simulink model "WaterTank_10Tanks_Model"  (R2013a)
settings: Solver=ode3  StartTime=0.0  StopTime=30.0  FixedStep=0.001  RelTol=1e-3
InitFcn:
  | initparametersDACADC
undefined symbols (not defined in the file): Ad, Bd, Cd, Dd, x0
libraries: commutil2 x1080, xpclib x142, etargetslib x140, dspnetwork x140, commcrc2 x20, simulink x1
(part 3 of 9)

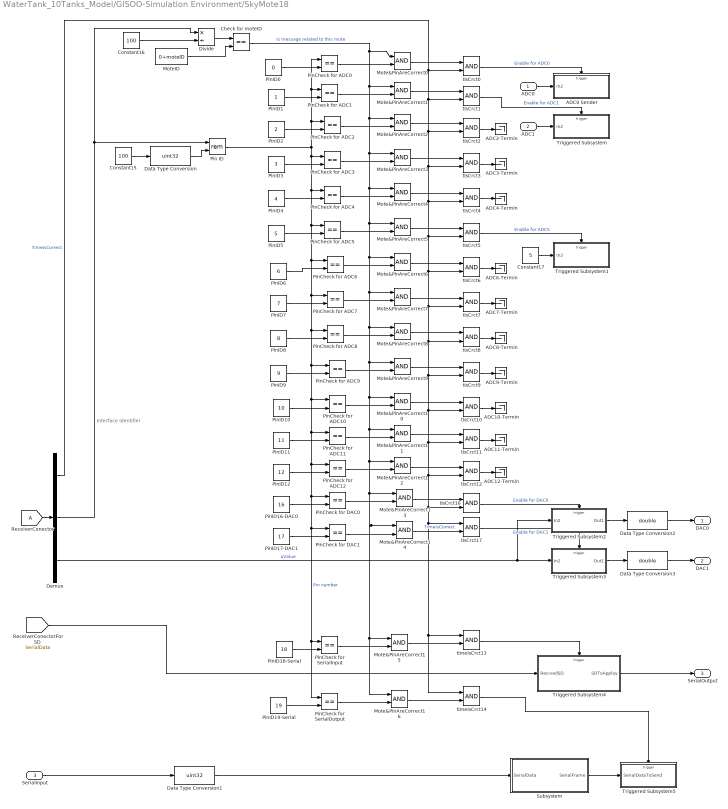
== system WaterTank_10Tanks_Model/GISOO-Simulation Environment/SkyMote18 ==
  note: Interface Identifier
  ADC0 : Inport
  ADC1 : Inport  Port=2
  SerialInput : Inport  Port=3
  ADC0 Sender : Subsystem  TreatAsAtomicUnit=on
  ADC10-Termin : Terminator
  ADC11-Termin : Terminator
  ADC12-Termin : Terminator
  ADC2-Termin : Terminator
  ADC3-Termin : Terminator
  ADC4-Termin : Terminator
  ADC6-Termin : Terminator
  ADC7-Termin : Terminator
  ADC8-Termin : Terminator
  ADC9-Termin : Terminator
  Check for moteID : RelationalOperator  Operator===  OutDataTypeStr=boolean
  Constant15 : Constant  Value=100
  Constant16 : Constant  Value=100
  Constant17 : Constant  Value=5
  Data Type Conversion : DataTypeConversion  OutDataTypeStr=uint32
  Data Type Conversion1 : DataTypeConversion  OutDataTypeStr=uint32
  Data Type Conversion2 : DataTypeConversion  OutDataTypeStr=double
  Data Type Conversion3 : DataTypeConversion  OutDataTypeStr=double
  Demux : Demux  Outputs=3
  Divide : Product  Inputs=*/  OutDataTypeStr=int32
  Mote&PinAreCorrect{0..16} (17 alike) : Logic  AllPortsSameDT=off  OutDataTypeStr=boolean
  MoteID : Constant  Value=0+moteID
  Pin ID : Math  Operator=rem  SaturateOnIntegerOverflow=on
  PinCheck for ADC{0..12} (13 alike) : RelationalOperator  Operator===  OutDataTypeStr=boolean
  PinCheck for DAC0 : RelationalOperator  Operator===  OutDataTypeStr=boolean
  PinCheck for DAC1 : RelationalOperator  Operator===  OutDataTypeStr=boolean
  PinCheck for SerialInput : RelationalOperator  Operator===  OutDataTypeStr=boolean
  PinCheck for SerialOutput : RelationalOperator  Operator===  OutDataTypeStr=boolean
  PinID0 : Constant  Value=0
  PinID1 : Constant
  PinID10 : Constant  Value=10
  PinID11 : Constant  Value=11
  PinID12 : Constant  Value=12
  PinID16-DAC0 : Constant  Value=16
  PinID17-DAC1 : Constant  Value=17
  PinID18-Serial : Constant  Value=18
  PinID19-Serial : Constant  Value=19
  PinID2 : Constant  Value=2
  PinID3 : Constant  Value=3
  PinID4 : Constant  Value=4
  PinID5 : Constant  Value=5
  PinID6 : Constant  Value=6
  PinID7 : Constant  Value=7
  PinID8 : Constant  Value=8
  PinID9 : Constant  Value=9
  Subsystem : Subsystem
  Triggered Subsystem : Subsystem  TreatAsAtomicUnit=on
  Triggered Subsystem1 : Subsystem  TreatAsAtomicUnit=on
  Triggered Subsystem2 : Subsystem  TreatAsAtomicUnit=on
  Triggered Subsystem3 : Subsystem  TreatAsAtomicUnit=on
  Triggered Subsystem4 : Subsystem  TreatAsAtomicUnit=on
  Triggered Subsystem5 : Subsystem  TreatAsAtomicUnit=on
  tIsCrct{0..12,16..17} (15 alike) : Logic  AllPortsSameDT=off  OutDataTypeStr=boolean
  timeIsCrct13 : Logic  AllPortsSameDT=off  OutDataTypeStr=boolean
  timeIsCrct14 : Logic  AllPortsSameDT=off  OutDataTypeStr=boolean
  DAC0 : Outport
  DAC1 : Outport  Port=2
  SerialOutput : Outport  Port=3
  wires:
  PinCheck for SerialInput/1 -> Mote&PinAreCorrect15/2
  Data Type Conversion1/1 -> Subsystem/1(SerialData)
  SerialInput/1 -> Data Type Conversion1/1
  timeIsCrct14/1 -> Triggered Subsystem5/Trigger
  Mote&PinAreCorrect16/1 -> timeIsCrct14/2
  PinCheck for SerialOutput/1 -> Mote&PinAreCorrect16/2
  PinID19-Serial/1 -> PinCheck for SerialOutput/2
  Check for moteID/1 -> Mote&PinAreCorrect0/1, Mote&PinAreCorrect2/1, Mote&PinAreCorrect3/1, Mote&PinAreCorrect4/1, Mote&PinAreCorrect5/1, Mote&PinAreCorrect6/1, Mote&PinAreCorrect7/1, Mote&PinAreCorrect8/1, Mote&PinAreCorrect9/1, Mote&PinAreCorrect10/1, Mote&PinAreCorrect11/1, Mote&PinAreCorrect12/1, Mote&PinAreCorrect15/1, Mote&PinAreCorrect16/1, Mote&PinAreCorrect14/1, Mote&PinAreCorrect13/1, Mote&PinAreCorrect1/1  "Is message related to this mote"
  Mote&PinAreCorrect15/1 -> timeIsCrct13/2
  Pin ID/1 -> PinCheck for ADC3/1, PinCheck for ADC4/1, PinCheck for ADC5/1, PinCheck for ADC6/1, PinCheck for ADC7/1, PinCheck for ADC8/1, PinCheck for ADC9/1, PinCheck for ADC10/1, PinCheck for ADC11/1, PinCheck for ADC12/1, PinCheck for DAC0/1, PinCheck for DAC1/1, PinCheck for SerialInput/1, PinCheck for SerialOutput/1, PinCheck for ADC2/1, PinCheck for ADC1/1, PinCheck for ADC0/1  "Pin number"
  tIsCrct12/1 -> ADC12-Termin/1
  Triggered Subsystem4/1(SDToApplay) -> SerialOutput/1
  Mote&PinAreCorrect14/1 -> tIsCrct17/2  "TimeIsCorrect"
  timeIsCrct13/1 -> Triggered Subsystem4/Trigger
  [SerialData] -> Triggered Subsystem4/1(RecivedSD)
  PinID18-Serial/1 -> PinCheck for SerialInput/2
  Demux/1 -> tIsCrct17/1, timeIsCrct13/1, timeIsCrct14/1, tIsCrct16/2, tIsCrct12/2, tIsCrct11/2, tIsCrct10/2, tIsCrct9/2, tIsCrct8/2, tIsCrct7/2, tIsCrct6/2, tIsCrct5/2, tIsCrct4/2, tIsCrct3/2, tIsCrct2/2, tIsCrct1/2, tIsCrct0/2  "TimeIsCorrect"
  Subsystem/1(SerialFrame) -> Triggered Subsystem5/1(SerialDataToSend)
  PinID17-DAC1/1 -> PinCheck for DAC1/2
  PinID16-DAC0/1 -> PinCheck for DAC0/2
  PinID12/1 -> PinCheck for ADC12/2
  PinID11/1 -> PinCheck for ADC11/2
  PinID9/1 -> PinCheck for ADC9/2
  PinID1/1 -> PinCheck for ADC1/2
  PinID10/1 -> PinCheck for ADC10/2
  PinID8/1 -> PinCheck for ADC8/2
  PinID7/1 -> PinCheck for ADC7/2
  PinID6/1 -> PinCheck for ADC6/2
  PinID5/1 -> PinCheck for ADC5/2
  PinID4/1 -> PinCheck for ADC4/2
  PinID3/1 -> PinCheck for ADC3/2
  PinID2/1 -> PinCheck for ADC2/2
  PinID0/1 -> PinCheck for ADC0/2
  PinCheck for ADC0/1 -> Mote&PinAreCorrect0/2
  PinCheck for ADC1/1 -> Mote&PinAreCorrect1/2
  PinCheck for ADC2/1 -> Mote&PinAreCorrect2/2
  PinCheck for ADC3/1 -> Mote&PinAreCorrect3/2
  PinCheck for ADC4/1 -> Mote&PinAreCorrect4/2
  PinCheck for ADC5/1 -> Mote&PinAreCorrect5/2
  PinCheck for ADC6/1 -> Mote&PinAreCorrect6/2
  PinCheck for ADC7/1 -> Mote&PinAreCorrect7/2
  PinCheck for ADC8/1 -> Mote&PinAreCorrect8/2
  PinCheck for ADC9/1 -> Mote&PinAreCorrect9/2
  PinCheck for ADC10/1 -> Mote&PinAreCorrect10/2
  PinCheck for ADC11/1 -> Mote&PinAreCorrect11/2
  PinCheck for ADC12/1 -> Mote&PinAreCorrect12/2
  PinCheck for DAC0/1 -> Mote&PinAreCorrect13/2
  PinCheck for DAC1/1 -> Mote&PinAreCorrect14/2
  Constant16/1 -> Divide/2
  Divide/1 -> Check for moteID/1
  MoteID/1 -> Check for moteID/2
  Mote&PinAreCorrect13/1 -> tIsCrct16/1
  Mote&PinAreCorrect12/1 -> tIsCrct12/1
  Mote&PinAreCorrect8/1 -> tIsCrct8/1
  Mote&PinAreCorrect7/1 -> tIsCrct7/1
  Mote&PinAreCorrect6/1 -> tIsCrct6/1
  Mote&PinAreCorrect4/1 -> tIsCrct4/1
  Mote&PinAreCorrect3/1 -> tIsCrct3/1
  Constant15/1 -> Data Type Conversion/1
  Data Type Conversion/1 -> Pin ID/2
  tIsCrct16/1 -> Triggered Subsystem2/Trigger  "Enable for DAC0"
  tIsCrct17/1 -> Triggered Subsystem3/Trigger  "Enable for DAC1"
  [A] -> Demux/1
  Demux/3 -> Triggered Subsystem3/1(In2), Triggered Subsystem2/1(In2)  "uValue"
  ADC0/1 -> ADC0 Sender/1(In2)
  Demux/2 -> Divide/1, Pin ID/1
  Data Type Conversion2/1 -> DAC0/1
  Triggered Subsystem2/1(Out1) -> Data Type Conversion2/1
  Data Type Conversion3/1 -> DAC1/1
  Triggered Subsystem3/1(Out1) -> Data Type Conversion3/1
  Constant17/1 -> Triggered Subsystem1/1(In2)
  Mote&PinAreCorrect0/1 -> tIsCrct0/1
  tIsCrct0/1 -> ADC0 Sender/Trigger  "Enable for ADC0"
  ADC1/1 -> Triggered Subsystem/1(In2)
  Mote&PinAreCorrect1/1 -> tIsCrct1/1
  tIsCrct1/1 -> Triggered Subsystem/Trigger  "Enable for ADC1"
  tIsCrct2/1 -> ADC2-Termin/1
  Mote&PinAreCorrect2/1 -> tIsCrct2/1
  tIsCrct3/1 -> ADC3-Termin/1
  tIsCrct4/1 -> ADC4-Termin/1
  tIsCrct6/1 -> ADC6-Termin/1
  Mote&PinAreCorrect5/1 -> tIsCrct5/1
  tIsCrct5/1 -> Triggered Subsystem1/Trigger  "Enable for ADC5"
  tIsCrct7/1 -> ADC7-Termin/1
  tIsCrct8/1 -> ADC8-Termin/1
  tIsCrct9/1 -> ADC9-Termin/1
  Mote&PinAreCorrect9/1 -> tIsCrct9/1
  tIsCrct10/1 -> ADC10-Termin/1
  Mote&PinAreCorrect10/1 -> tIsCrct10/1
  tIsCrct11/1 -> ADC11-Termin/1
  Mote&PinAreCorrect11/1 -> tIsCrct11/1

== system WaterTank_10Tanks_Model/GISOO-Simulation Environment/SkyMote19 ==
  note: Interface Identifier
  ADC0 : Inport
  ADC1 : Inport  Port=2
  SerialInput : Inport  Port=3
  ADC0 Sender : Subsystem  TreatAsAtomicUnit=on
  ADC10-Termin : Terminator
  ADC11-Termin : Terminator
  ADC12-Termin : Terminator
  ADC2-Termin : Terminator
  ADC3-Termin : Terminator
  ADC4-Termin : Terminator
  ADC6-Termin : Terminator
  ADC7-Termin : Terminator
  ADC8-Termin : Terminator
  ADC9-Termin : Terminator
  Check for moteID : RelationalOperator  Operator===  OutDataTypeStr=boolean
  Constant15 : Constant  Value=100
  Constant16 : Constant  Value=100
  Constant17 : Constant  Value=5
  Data Type Conversion : DataTypeConversion  OutDataTypeStr=uint32
  Data Type Conversion1 : DataTypeConversion  OutDataTypeStr=uint32
  Data Type Conversion2 : DataTypeConversion  OutDataTypeStr=double
  Data Type Conversion3 : DataTypeConversion  OutDataTypeStr=double
  Demux : Demux  Outputs=3
  Divide : Product  Inputs=*/  OutDataTypeStr=int32
  Mote&PinAreCorrect{0..16} (17 alike) : Logic  AllPortsSameDT=off  OutDataTypeStr=boolean
  MoteID : Constant  Value=0+moteID
  Pin ID : Math  Operator=rem  SaturateOnIntegerOverflow=on
  PinCheck for ADC{0..12} (13 alike) : RelationalOperator  Operator===  OutDataTypeStr=boolean
  PinCheck for DAC0 : RelationalOperator  Operator===  OutDataTypeStr=boolean
  PinCheck for DAC1 : RelationalOperator  Operator===  OutDataTypeStr=boolean
  PinCheck for SerialInput : RelationalOperator  Operator===  OutDataTypeStr=boolean
  PinCheck for SerialOutput : RelationalOperator  Operator===  OutDataTypeStr=boolean
  PinID0 : Constant  Value=0
  PinID1 : Constant
  PinID10 : Constant  Value=10
  PinID11 : Constant  Value=11
  PinID12 : Constant  Value=12
  PinID16-DAC0 : Constant  Value=16
  PinID17-DAC1 : Constant  Value=17
  PinID18-Serial : Constant  Value=18
  PinID19-Serial : Constant  Value=19
  PinID2 : Constant  Value=2
  PinID3 : Constant  Value=3
  PinID4 : Constant  Value=4
  PinID5 : Constant  Value=5
  PinID6 : Constant  Value=6
  PinID7 : Constant  Value=7
  PinID8 : Constant  Value=8
  PinID9 : Constant  Value=9
  Subsystem : Subsystem
  Triggered Subsystem : Subsystem  TreatAsAtomicUnit=on
  Triggered Subsystem1 : Subsystem  TreatAsAtomicUnit=on
  Triggered Subsystem2 : Subsystem  TreatAsAtomicUnit=on
  Triggered Subsystem3 : Subsystem  TreatAsAtomicUnit=on
  Triggered Subsystem4 : Subsystem  TreatAsAtomicUnit=on
  Triggered Subsystem5 : Subsystem  TreatAsAtomicUnit=on
  tIsCrct{0..12,16..17} (15 alike) : Logic  AllPortsSameDT=off  OutDataTypeStr=boolean
  timeIsCrct13 : Logic  AllPortsSameDT=off  OutDataTypeStr=boolean
  timeIsCrct14 : Logic  AllPortsSameDT=off  OutDataTypeStr=boolean
  DAC0 : Outport
  DAC1 : Outport  Port=2
  SerialOutput : Outport  Port=3
  wires:
  Mote&PinAreCorrect11/1 -> tIsCrct11/1
  tIsCrct11/1 -> ADC11-Termin/1
  Mote&PinAreCorrect10/1 -> tIsCrct10/1
  tIsCrct10/1 -> ADC10-Termin/1
  Mote&PinAreCorrect9/1 -> tIsCrct9/1
  tIsCrct9/1 -> ADC9-Termin/1
  tIsCrct8/1 -> ADC8-Termin/1
  tIsCrct7/1 -> ADC7-Termin/1
  tIsCrct5/1 -> Triggered Subsystem1/Trigger  "Enable for ADC5"
  Mote&PinAreCorrect5/1 -> tIsCrct5/1
  tIsCrct6/1 -> ADC6-Termin/1
  tIsCrct4/1 -> ADC4-Termin/1
  tIsCrct3/1 -> ADC3-Termin/1
  Mote&PinAreCorrect2/1 -> tIsCrct2/1
  tIsCrct2/1 -> ADC2-Termin/1
  tIsCrct1/1 -> Triggered Subsystem/Trigger  "Enable for ADC1"
  Mote&PinAreCorrect1/1 -> tIsCrct1/1
  ADC1/1 -> Triggered Subsystem/1(In2)
  tIsCrct0/1 -> ADC0 Sender/Trigger  "Enable for ADC0"
  Mote&PinAreCorrect0/1 -> tIsCrct0/1
  Constant17/1 -> Triggered Subsystem1/1(In2)
  Triggered Subsystem3/1(Out1) -> Data Type Conversion3/1
  Data Type Conversion3/1 -> DAC1/1
  Triggered Subsystem2/1(Out1) -> Data Type Conversion2/1
  Data Type Conversion2/1 -> DAC0/1
  Demux/2 -> Pin ID/1, Divide/1
  ADC0/1 -> ADC0 Sender/1(In2)
  Demux/3 -> Triggered Subsystem2/1(In2), Triggered Subsystem3/1(In2)  "uValue"
  [A] -> Demux/1
  tIsCrct17/1 -> Triggered Subsystem3/Trigger  "Enable for DAC1"
  tIsCrct16/1 -> Triggered Subsystem2/Trigger  "Enable for DAC0"
  Data Type Conversion/1 -> Pin ID/2
  Constant15/1 -> Data Type Conversion/1
  Mote&PinAreCorrect3/1 -> tIsCrct3/1
  Mote&PinAreCorrect4/1 -> tIsCrct4/1
  Mote&PinAreCorrect6/1 -> tIsCrct6/1
  Mote&PinAreCorrect7/1 -> tIsCrct7/1
  Mote&PinAreCorrect8/1 -> tIsCrct8/1
  Mote&PinAreCorrect12/1 -> tIsCrct12/1
  Mote&PinAreCorrect13/1 -> tIsCrct16/1
  MoteID/1 -> Check for moteID/2
  Divide/1 -> Check for moteID/1
  Constant16/1 -> Divide/2
  PinCheck for DAC1/1 -> Mote&PinAreCorrect14/2
  PinCheck for DAC0/1 -> Mote&PinAreCorrect13/2
  PinCheck for ADC12/1 -> Mote&PinAreCorrect12/2
  PinCheck for ADC11/1 -> Mote&PinAreCorrect11/2
  PinCheck for ADC10/1 -> Mote&PinAreCorrect10/2
  PinCheck for ADC9/1 -> Mote&PinAreCorrect9/2
  PinCheck for ADC8/1 -> Mote&PinAreCorrect8/2
  PinCheck for ADC7/1 -> Mote&PinAreCorrect7/2
  PinCheck for ADC6/1 -> Mote&PinAreCorrect6/2
  PinCheck for ADC5/1 -> Mote&PinAreCorrect5/2
  PinCheck for ADC4/1 -> Mote&PinAreCorrect4/2
  PinCheck for ADC3/1 -> Mote&PinAreCorrect3/2
  PinCheck for ADC2/1 -> Mote&PinAreCorrect2/2
  PinCheck for ADC1/1 -> Mote&PinAreCorrect1/2
  PinCheck for ADC0/1 -> Mote&PinAreCorrect0/2
  PinID0/1 -> PinCheck for ADC0/2
  PinID2/1 -> PinCheck for ADC2/2
  PinID3/1 -> PinCheck for ADC3/2
  PinID4/1 -> PinCheck for ADC4/2
  PinID5/1 -> PinCheck for ADC5/2
  PinID6/1 -> PinCheck for ADC6/2
  PinID7/1 -> PinCheck for ADC7/2
  PinID8/1 -> PinCheck for ADC8/2
  PinID10/1 -> PinCheck for ADC10/2
  PinID1/1 -> PinCheck for ADC1/2
  PinID9/1 -> PinCheck for ADC9/2
  PinID11/1 -> PinCheck for ADC11/2
  PinID12/1 -> PinCheck for ADC12/2
  PinID16-DAC0/1 -> PinCheck for DAC0/2
  PinID17-DAC1/1 -> PinCheck for DAC1/2
  Subsystem/1(SerialFrame) -> Triggered Subsystem5/1(SerialDataToSend)
  Demux/1 -> tIsCrct0/2, tIsCrct1/2, tIsCrct2/2, tIsCrct3/2, tIsCrct4/2, tIsCrct5/2, tIsCrct6/2, tIsCrct7/2, tIsCrct8/2, tIsCrct9/2, tIsCrct10/2, tIsCrct11/2, tIsCrct12/2, tIsCrct16/2, timeIsCrct14/1, timeIsCrct13/1, tIsCrct17/1  "TimeIsCorrect"
  PinID18-Serial/1 -> PinCheck for SerialInput/2
  [SerialData] -> Triggered Subsystem4/1(RecivedSD)
  timeIsCrct13/1 -> Triggered Subsystem4/Trigger
  Mote&PinAreCorrect14/1 -> tIsCrct17/2  "TimeIsCorrect"
  Triggered Subsystem4/1(SDToApplay) -> SerialOutput/1
  tIsCrct12/1 -> ADC12-Termin/1
  Pin ID/1 -> PinCheck for ADC0/1, PinCheck for ADC1/1, PinCheck for ADC2/1, PinCheck for SerialOutput/1, PinCheck for SerialInput/1, PinCheck for DAC1/1, PinCheck for DAC0/1, PinCheck for ADC12/1, PinCheck for ADC11/1, PinCheck for ADC10/1, PinCheck for ADC9/1, PinCheck for ADC8/1, PinCheck for ADC7/1, PinCheck for ADC6/1, PinCheck for ADC5/1, PinCheck for ADC4/1, PinCheck for ADC3/1  "Pin number"
  Mote&PinAreCorrect15/1 -> timeIsCrct13/2
  Check for moteID/1 -> Mote&PinAreCorrect1/1, Mote&PinAreCorrect13/1, Mote&PinAreCorrect14/1, Mote&PinAreCorrect16/1, Mote&PinAreCorrect15/1, Mote&PinAreCorrect12/1, Mote&PinAreCorrect11/1, Mote&PinAreCorrect10/1, Mote&PinAreCorrect9/1, Mote&PinAreCorrect8/1, Mote&PinAreCorrect7/1, Mote&PinAreCorrect6/1, Mote&PinAreCorrect5/1, Mote&PinAreCorrect4/1, Mote&PinAreCorrect3/1, Mote&PinAreCorrect2/1, Mote&PinAreCorrect0/1  "Is message related to this mote"
  PinID19-Serial/1 -> PinCheck for SerialOutput/2
  PinCheck for SerialOutput/1 -> Mote&PinAreCorrect16/2
  Mote&PinAreCorrect16/1 -> timeIsCrct14/2
  timeIsCrct14/1 -> Triggered Subsystem5/Trigger
  SerialInput/1 -> Data Type Conversion1/1
  Data Type Conversion1/1 -> Subsystem/1(SerialData)
  PinCheck for SerialInput/1 -> Mote&PinAreCorrect15/2

== system WaterTank_10Tanks_Model/GISOO-Simulation Environment/SkyMote2 ==
  note: Interface Identifier
  ADC0 : Inport
  ADC1 : Inport  Port=2
  SerialInput : Inport  Port=3
  ADC0 Sender : Subsystem  TreatAsAtomicUnit=on
  ADC10-Termin : Terminator
  ADC11-Termin : Terminator
  ADC12-Termin : Terminator
  ADC2-Termin : Terminator
  ADC3-Termin : Terminator
  ADC4-Termin : Terminator
  ADC6-Termin : Terminator
  ADC7-Termin : Terminator
  ADC8-Termin : Terminator
  ADC9-Termin : Terminator
  Check for moteID : RelationalOperator  Operator===  OutDataTypeStr=boolean
  Constant15 : Constant  Value=100
  Constant16 : Constant  Value=100
  Constant17 : Constant  Value=5
  Data Type Conversion : DataTypeConversion  OutDataTypeStr=uint32
  Data Type Conversion1 : DataTypeConversion  OutDataTypeStr=uint32
  Data Type Conversion2 : DataTypeConversion  OutDataTypeStr=double
  Data Type Conversion3 : DataTypeConversion  OutDataTypeStr=double
  Demux : Demux  Outputs=3
  Divide : Product  Inputs=*/  OutDataTypeStr=int32
  Mote&PinAreCorrect{0..16} (17 alike) : Logic  AllPortsSameDT=off  OutDataTypeStr=boolean
  MoteID : Constant  Value=0+moteID
  Pin ID : Math  Operator=rem  SaturateOnIntegerOverflow=on
  PinCheck for ADC{0..12} (13 alike) : RelationalOperator  Operator===  OutDataTypeStr=boolean
  PinCheck for DAC0 : RelationalOperator  Operator===  OutDataTypeStr=boolean
  PinCheck for DAC1 : RelationalOperator  Operator===  OutDataTypeStr=boolean
  PinCheck for SerialInput : RelationalOperator  Operator===  OutDataTypeStr=boolean
  PinCheck for SerialOutput : RelationalOperator  Operator===  OutDataTypeStr=boolean
  PinID0 : Constant  Value=0
  PinID1 : Constant
  PinID10 : Constant  Value=10
  PinID11 : Constant  Value=11
  PinID12 : Constant  Value=12
  PinID16-DAC0 : Constant  Value=16
  PinID17-DAC1 : Constant  Value=17
  PinID18-Serial : Constant  Value=18
  PinID19-Serial : Constant  Value=19
  PinID2 : Constant  Value=2
  PinID3 : Constant  Value=3
  PinID4 : Constant  Value=4
  PinID5 : Constant  Value=5
  PinID6 : Constant  Value=6
  PinID7 : Constant  Value=7
  PinID8 : Constant  Value=8
  PinID9 : Constant  Value=9
  Subsystem : Subsystem
  Triggered Subsystem : Subsystem  TreatAsAtomicUnit=on
  Triggered Subsystem1 : Subsystem  TreatAsAtomicUnit=on
  Triggered Subsystem2 : Subsystem  TreatAsAtomicUnit=on
  Triggered Subsystem3 : Subsystem  TreatAsAtomicUnit=on
  Triggered Subsystem4 : Subsystem  TreatAsAtomicUnit=on
  Triggered Subsystem5 : Subsystem  TreatAsAtomicUnit=on
  tIsCrct{0..12,16..17} (15 alike) : Logic  AllPortsSameDT=off  OutDataTypeStr=boolean
  timeIsCrct13 : Logic  AllPortsSameDT=off  OutDataTypeStr=boolean
  timeIsCrct14 : Logic  AllPortsSameDT=off  OutDataTypeStr=boolean
  DAC0 : Outport
  DAC1 : Outport  Port=2
  SerialOutput : Outport  Port=3
  wires:
  PinCheck for SerialInput/1 -> Mote&PinAreCorrect15/2
  Data Type Conversion1/1 -> Subsystem/1(SerialData)
  SerialInput/1 -> Data Type Conversion1/1
  timeIsCrct14/1 -> Triggered Subsystem5/Trigger
  Mote&PinAreCorrect16/1 -> timeIsCrct14/2
  PinCheck for SerialOutput/1 -> Mote&PinAreCorrect16/2
  PinID19-Serial/1 -> PinCheck for SerialOutput/2
  Check for moteID/1 -> Mote&PinAreCorrect0/1, Mote&PinAreCorrect2/1, Mote&PinAreCorrect3/1, Mote&PinAreCorrect4/1, Mote&PinAreCorrect5/1, Mote&PinAreCorrect6/1, Mote&PinAreCorrect7/1, Mote&PinAreCorrect8/1, Mote&PinAreCorrect9/1, Mote&PinAreCorrect10/1, Mote&PinAreCorrect11/1, Mote&PinAreCorrect12/1, Mote&PinAreCorrect15/1, Mote&PinAreCorrect16/1, Mote&PinAreCorrect14/1, Mote&PinAreCorrect13/1, Mote&PinAreCorrect1/1  "Is message related to this mote"
  Mote&PinAreCorrect15/1 -> timeIsCrct13/2
  Pin ID/1 -> PinCheck for ADC3/1, PinCheck for ADC4/1, PinCheck for ADC5/1, PinCheck for ADC6/1, PinCheck for ADC7/1, PinCheck for ADC8/1, PinCheck for ADC9/1, PinCheck for ADC10/1, PinCheck for ADC11/1, PinCheck for ADC12/1, PinCheck for DAC0/1, PinCheck for DAC1/1, PinCheck for SerialInput/1, PinCheck for SerialOutput/1, PinCheck for ADC2/1, PinCheck for ADC1/1, PinCheck for ADC0/1  "Pin number"
  tIsCrct12/1 -> ADC12-Termin/1
  Triggered Subsystem4/1(SDToApplay) -> SerialOutput/1
  Mote&PinAreCorrect14/1 -> tIsCrct17/2  "TimeIsCorrect"
  timeIsCrct13/1 -> Triggered Subsystem4/Trigger
  [SerialData] -> Triggered Subsystem4/1(RecivedSD)
  PinID18-Serial/1 -> PinCheck for SerialInput/2
  Demux/1 -> tIsCrct17/1, timeIsCrct13/1, timeIsCrct14/1, tIsCrct16/2, tIsCrct12/2, tIsCrct11/2, tIsCrct10/2, tIsCrct9/2, tIsCrct8/2, tIsCrct7/2, tIsCrct6/2, tIsCrct5/2, tIsCrct4/2, tIsCrct3/2, tIsCrct2/2, tIsCrct1/2, tIsCrct0/2  "TimeIsCorrect"
  Subsystem/1(SerialFrame) -> Triggered Subsystem5/1(SerialDataToSend)
  PinID17-DAC1/1 -> PinCheck for DAC1/2
  PinID16-DAC0/1 -> PinCheck for DAC0/2
  PinID12/1 -> PinCheck for ADC12/2
  PinID11/1 -> PinCheck for ADC11/2
  PinID9/1 -> PinCheck for ADC9/2
  PinID1/1 -> PinCheck for ADC1/2
  PinID10/1 -> PinCheck for ADC10/2
  PinID8/1 -> PinCheck for ADC8/2
  PinID7/1 -> PinCheck for ADC7/2
  PinID6/1 -> PinCheck for ADC6/2
  PinID5/1 -> PinCheck for ADC5/2
  PinID4/1 -> PinCheck for ADC4/2
  PinID3/1 -> PinCheck for ADC3/2
  PinID2/1 -> PinCheck for ADC2/2
  PinID0/1 -> PinCheck for ADC0/2
  PinCheck for ADC0/1 -> Mote&PinAreCorrect0/2
  PinCheck for ADC1/1 -> Mote&PinAreCorrect1/2
  PinCheck for ADC2/1 -> Mote&PinAreCorrect2/2
  PinCheck for ADC3/1 -> Mote&PinAreCorrect3/2
  PinCheck for ADC4/1 -> Mote&PinAreCorrect4/2
  PinCheck for ADC5/1 -> Mote&PinAreCorrect5/2
  PinCheck for ADC6/1 -> Mote&PinAreCorrect6/2
  PinCheck for ADC7/1 -> Mote&PinAreCorrect7/2
  PinCheck for ADC8/1 -> Mote&PinAreCorrect8/2
  PinCheck for ADC9/1 -> Mote&PinAreCorrect9/2
  PinCheck for ADC10/1 -> Mote&PinAreCorrect10/2
  PinCheck for ADC11/1 -> Mote&PinAreCorrect11/2
  PinCheck for ADC12/1 -> Mote&PinAreCorrect12/2
  PinCheck for DAC0/1 -> Mote&PinAreCorrect13/2
  PinCheck for DAC1/1 -> Mote&PinAreCorrect14/2
  Constant16/1 -> Divide/2
  Divide/1 -> Check for moteID/1
  MoteID/1 -> Check for moteID/2
  Mote&PinAreCorrect13/1 -> tIsCrct16/1
  Mote&PinAreCorrect12/1 -> tIsCrct12/1
  Mote&PinAreCorrect8/1 -> tIsCrct8/1
  Mote&PinAreCorrect7/1 -> tIsCrct7/1
  Mote&PinAreCorrect6/1 -> tIsCrct6/1
  Mote&PinAreCorrect4/1 -> tIsCrct4/1
  Mote&PinAreCorrect3/1 -> tIsCrct3/1
  Constant15/1 -> Data Type Conversion/1
  Data Type Conversion/1 -> Pin ID/2
  tIsCrct16/1 -> Triggered Subsystem2/Trigger  "Enable for DAC0"
  tIsCrct17/1 -> Triggered Subsystem3/Trigger  "Enable for DAC1"
  [A] -> Demux/1
  Demux/3 -> Triggered Subsystem3/1(In2), Triggered Subsystem2/1(In2)  "uValue"
  ADC0/1 -> ADC0 Sender/1(In2)
  Demux/2 -> Divide/1, Pin ID/1
  Data Type Conversion2/1 -> DAC0/1
  Triggered Subsystem2/1(Out1) -> Data Type Conversion2/1
  Data Type Conversion3/1 -> DAC1/1
  Triggered Subsystem3/1(Out1) -> Data Type Conversion3/1
  Constant17/1 -> Triggered Subsystem1/1(In2)
  Mote&PinAreCorrect0/1 -> tIsCrct0/1
  tIsCrct0/1 -> ADC0 Sender/Trigger  "Enable for ADC0"
  ADC1/1 -> Triggered Subsystem/1(In2)
  Mote&PinAreCorrect1/1 -> tIsCrct1/1
  tIsCrct1/1 -> Triggered Subsystem/Trigger  "Enable for ADC1"
  tIsCrct2/1 -> ADC2-Termin/1
  Mote&PinAreCorrect2/1 -> tIsCrct2/1
  tIsCrct3/1 -> ADC3-Termin/1
  tIsCrct4/1 -> ADC4-Termin/1
  tIsCrct6/1 -> ADC6-Termin/1
  Mote&PinAreCorrect5/1 -> tIsCrct5/1
  tIsCrct5/1 -> Triggered Subsystem1/Trigger  "Enable for ADC5"
  tIsCrct7/1 -> ADC7-Termin/1
  tIsCrct8/1 -> ADC8-Termin/1
  tIsCrct9/1 -> ADC9-Termin/1
  Mote&PinAreCorrect9/1 -> tIsCrct9/1
  tIsCrct10/1 -> ADC10-Termin/1
  Mote&PinAreCorrect10/1 -> tIsCrct10/1
  tIsCrct11/1 -> ADC11-Termin/1
  Mote&PinAreCorrect11/1 -> tIsCrct11/1

== system WaterTank_10Tanks_Model/GISOO-Simulation Environment/SkyMote3 ==
  note: Interface Identifier
  ADC0 : Inport
  ADC1 : Inport  Port=2
  SerialInput : Inport  Port=3
  ADC0 Sender : Subsystem  TreatAsAtomicUnit=on
  ADC10-Termin : Terminator
  ADC11-Termin : Terminator
  ADC12-Termin : Terminator
  ADC2-Termin : Terminator
  ADC3-Termin : Terminator
  ADC4-Termin : Terminator
  ADC6-Termin : Terminator
  ADC7-Termin : Terminator
  ADC8-Termin : Terminator
  ADC9-Termin : Terminator
  Check for moteID : RelationalOperator  Operator===  OutDataTypeStr=boolean
  Constant15 : Constant  Value=100
  Constant16 : Constant  Value=100
  Constant17 : Constant  Value=5
  Data Type Conversion : DataTypeConversion  OutDataTypeStr=uint32
  Data Type Conversion1 : DataTypeConversion  OutDataTypeStr=uint32
  Data Type Conversion2 : DataTypeConversion  OutDataTypeStr=double
  Data Type Conversion3 : DataTypeConversion  OutDataTypeStr=double
  Demux : Demux  Outputs=3
  Divide : Product  Inputs=*/  OutDataTypeStr=int32
  Mote&PinAreCorrect{0..16} (17 alike) : Logic  AllPortsSameDT=off  OutDataTypeStr=boolean
  MoteID : Constant  Value=0+moteID
  Pin ID : Math  Operator=rem  SaturateOnIntegerOverflow=on
  PinCheck for ADC{0..12} (13 alike) : RelationalOperator  Operator===  OutDataTypeStr=boolean
  PinCheck for DAC0 : RelationalOperator  Operator===  OutDataTypeStr=boolean
  PinCheck for DAC1 : RelationalOperator  Operator===  OutDataTypeStr=boolean
  PinCheck for SerialInput : RelationalOperator  Operator===  OutDataTypeStr=boolean
  PinCheck for SerialOutput : RelationalOperator  Operator===  OutDataTypeStr=boolean
  PinID0 : Constant  Value=0
  PinID1 : Constant
  PinID10 : Constant  Value=10
  PinID11 : Constant  Value=11
  PinID12 : Constant  Value=12
  PinID16-DAC0 : Constant  Value=16
  PinID17-DAC1 : Constant  Value=17
  PinID18-Serial : Constant  Value=18
  PinID19-Serial : Constant  Value=19
  PinID2 : Constant  Value=2
  PinID3 : Constant  Value=3
  PinID4 : Constant  Value=4
  PinID5 : Constant  Value=5
  PinID6 : Constant  Value=6
  PinID7 : Constant  Value=7
  PinID8 : Constant  Value=8
  PinID9 : Constant  Value=9
  Subsystem : Subsystem
  Triggered Subsystem : Subsystem  TreatAsAtomicUnit=on
  Triggered Subsystem1 : Subsystem  TreatAsAtomicUnit=on
  Triggered Subsystem2 : Subsystem  TreatAsAtomicUnit=on
  Triggered Subsystem3 : Subsystem  TreatAsAtomicUnit=on
  Triggered Subsystem4 : Subsystem  TreatAsAtomicUnit=on
  Triggered Subsystem5 : Subsystem  TreatAsAtomicUnit=on
  tIsCrct{0..12,16..17} (15 alike) : Logic  AllPortsSameDT=off  OutDataTypeStr=boolean
  timeIsCrct13 : Logic  AllPortsSameDT=off  OutDataTypeStr=boolean
  timeIsCrct14 : Logic  AllPortsSameDT=off  OutDataTypeStr=boolean
  DAC0 : Outport
  DAC1 : Outport  Port=2
  SerialOutput : Outport  Port=3
  wires:
  Mote&PinAreCorrect11/1 -> tIsCrct11/1
  tIsCrct11/1 -> ADC11-Termin/1
  Mote&PinAreCorrect10/1 -> tIsCrct10/1
  tIsCrct10/1 -> ADC10-Termin/1
  Mote&PinAreCorrect9/1 -> tIsCrct9/1
  tIsCrct9/1 -> ADC9-Termin/1
  tIsCrct8/1 -> ADC8-Termin/1
  tIsCrct7/1 -> ADC7-Termin/1
  tIsCrct5/1 -> Triggered Subsystem1/Trigger  "Enable for ADC5"
  Mote&PinAreCorrect5/1 -> tIsCrct5/1
  tIsCrct6/1 -> ADC6-Termin/1
  tIsCrct4/1 -> ADC4-Termin/1
  tIsCrct3/1 -> ADC3-Termin/1
  Mote&PinAreCorrect2/1 -> tIsCrct2/1
  tIsCrct2/1 -> ADC2-Termin/1
  tIsCrct1/1 -> Triggered Subsystem/Trigger  "Enable for ADC1"
  Mote&PinAreCorrect1/1 -> tIsCrct1/1
  ADC1/1 -> Triggered Subsystem/1(In2)
  tIsCrct0/1 -> ADC0 Sender/Trigger  "Enable for ADC0"
  Mote&PinAreCorrect0/1 -> tIsCrct0/1
  Constant17/1 -> Triggered Subsystem1/1(In2)
  Triggered Subsystem3/1(Out1) -> Data Type Conversion3/1
  Data Type Conversion3/1 -> DAC1/1
  Triggered Subsystem2/1(Out1) -> Data Type Conversion2/1
  Data Type Conversion2/1 -> DAC0/1
  Demux/2 -> Pin ID/1, Divide/1
  ADC0/1 -> ADC0 Sender/1(In2)
  Demux/3 -> Triggered Subsystem2/1(In2), Triggered Subsystem3/1(In2)  "uValue"
  [A] -> Demux/1
  tIsCrct17/1 -> Triggered Subsystem3/Trigger  "Enable for DAC1"
  tIsCrct16/1 -> Triggered Subsystem2/Trigger  "Enable for DAC0"
  Data Type Conversion/1 -> Pin ID/2
  Constant15/1 -> Data Type Conversion/1
  Mote&PinAreCorrect3/1 -> tIsCrct3/1
  Mote&PinAreCorrect4/1 -> tIsCrct4/1
  Mote&PinAreCorrect6/1 -> tIsCrct6/1
  Mote&PinAreCorrect7/1 -> tIsCrct7/1
  Mote&PinAreCorrect8/1 -> tIsCrct8/1
  Mote&PinAreCorrect12/1 -> tIsCrct12/1
  Mote&PinAreCorrect13/1 -> tIsCrct16/1
  MoteID/1 -> Check for moteID/2
  Divide/1 -> Check for moteID/1
  Constant16/1 -> Divide/2
  PinCheck for DAC1/1 -> Mote&PinAreCorrect14/2
  PinCheck for DAC0/1 -> Mote&PinAreCorrect13/2
  PinCheck for ADC12/1 -> Mote&PinAreCorrect12/2
  PinCheck for ADC11/1 -> Mote&PinAreCorrect11/2
  PinCheck for ADC10/1 -> Mote&PinAreCorrect10/2
  PinCheck for ADC9/1 -> Mote&PinAreCorrect9/2
  PinCheck for ADC8/1 -> Mote&PinAreCorrect8/2
  PinCheck for ADC7/1 -> Mote&PinAreCorrect7/2
  PinCheck for ADC6/1 -> Mote&PinAreCorrect6/2
  PinCheck for ADC5/1 -> Mote&PinAreCorrect5/2
  PinCheck for ADC4/1 -> Mote&PinAreCorrect4/2
  PinCheck for ADC3/1 -> Mote&PinAreCorrect3/2
  PinCheck for ADC2/1 -> Mote&PinAreCorrect2/2
  PinCheck for ADC1/1 -> Mote&PinAreCorrect1/2
  PinCheck for ADC0/1 -> Mote&PinAreCorrect0/2
  PinID0/1 -> PinCheck for ADC0/2
  PinID2/1 -> PinCheck for ADC2/2
  PinID3/1 -> PinCheck for ADC3/2
  PinID4/1 -> PinCheck for ADC4/2
  PinID5/1 -> PinCheck for ADC5/2
  PinID6/1 -> PinCheck for ADC6/2
  PinID7/1 -> PinCheck for ADC7/2
  PinID8/1 -> PinCheck for ADC8/2
  PinID10/1 -> PinCheck for ADC10/2
  PinID1/1 -> PinCheck for ADC1/2
  PinID9/1 -> PinCheck for ADC9/2
  PinID11/1 -> PinCheck for ADC11/2
  PinID12/1 -> PinCheck for ADC12/2
  PinID16-DAC0/1 -> PinCheck for DAC0/2
  PinID17-DAC1/1 -> PinCheck for DAC1/2
  Subsystem/1(SerialFrame) -> Triggered Subsystem5/1(SerialDataToSend)
  Demux/1 -> tIsCrct0/2, tIsCrct1/2, tIsCrct2/2, tIsCrct3/2, tIsCrct4/2, tIsCrct5/2, tIsCrct6/2, tIsCrct7/2, tIsCrct8/2, tIsCrct9/2, tIsCrct10/2, tIsCrct11/2, tIsCrct12/2, tIsCrct16/2, timeIsCrct14/1, timeIsCrct13/1, tIsCrct17/1  "TimeIsCorrect"
  PinID18-Serial/1 -> PinCheck for SerialInput/2
  [SerialData] -> Triggered Subsystem4/1(RecivedSD)
  timeIsCrct13/1 -> Triggered Subsystem4/Trigger
  Mote&PinAreCorrect14/1 -> tIsCrct17/2  "TimeIsCorrect"
  Triggered Subsystem4/1(SDToApplay) -> SerialOutput/1
  tIsCrct12/1 -> ADC12-Termin/1
  Pin ID/1 -> PinCheck for ADC0/1, PinCheck for ADC1/1, PinCheck for ADC2/1, PinCheck for SerialOutput/1, PinCheck for SerialInput/1, PinCheck for DAC1/1, PinCheck for DAC0/1, PinCheck for ADC12/1, PinCheck for ADC11/1, PinCheck for ADC10/1, PinCheck for ADC9/1, PinCheck for ADC8/1, PinCheck for ADC7/1, PinCheck for ADC6/1, PinCheck for ADC5/1, PinCheck for ADC4/1, PinCheck for ADC3/1  "Pin number"
  Mote&PinAreCorrect15/1 -> timeIsCrct13/2
  Check for moteID/1 -> Mote&PinAreCorrect1/1, Mote&PinAreCorrect13/1, Mote&PinAreCorrect14/1, Mote&PinAreCorrect16/1, Mote&PinAreCorrect15/1, Mote&PinAreCorrect12/1, Mote&PinAreCorrect11/1, Mote&PinAreCorrect10/1, Mote&PinAreCorrect9/1, Mote&PinAreCorrect8/1, Mote&PinAreCorrect7/1, Mote&PinAreCorrect6/1, Mote&PinAreCorrect5/1, Mote&PinAreCorrect4/1, Mote&PinAreCorrect3/1, Mote&PinAreCorrect2/1, Mote&PinAreCorrect0/1  "Is message related to this mote"
  PinID19-Serial/1 -> PinCheck for SerialOutput/2
  PinCheck for SerialOutput/1 -> Mote&PinAreCorrect16/2
  Mote&PinAreCorrect16/1 -> timeIsCrct14/2
  timeIsCrct14/1 -> Triggered Subsystem5/Trigger
  SerialInput/1 -> Data Type Conversion1/1
  Data Type Conversion1/1 -> Subsystem/1(SerialData)
  PinCheck for SerialInput/1 -> Mote&PinAreCorrect15/2

== system WaterTank_10Tanks_Model/GISOO-Simulation Environment/SkyMote4 ==
  note: Interface Identifier
  ADC0 : Inport
  ADC1 : Inport  Port=2
  SerialInput : Inport  Port=3
  ADC0 Sender : Subsystem  TreatAsAtomicUnit=on
  ADC10-Termin : Terminator
  ADC11-Termin : Terminator
  ADC12-Termin : Terminator
  ADC2-Termin : Terminator
  ADC3-Termin : Terminator
  ADC4-Termin : Terminator
  ADC6-Termin : Terminator
  ADC7-Termin : Terminator
  ADC8-Termin : Terminator
  ADC9-Termin : Terminator
  Check for moteID : RelationalOperator  Operator===  OutDataTypeStr=boolean
  Constant15 : Constant  Value=100
  Constant16 : Constant  Value=100
  Constant17 : Constant  Value=5
  Data Type Conversion : DataTypeConversion  OutDataTypeStr=uint32
  Data Type Conversion1 : DataTypeConversion  OutDataTypeStr=uint32
  Data Type Conversion2 : DataTypeConversion  OutDataTypeStr=double
  Data Type Conversion3 : DataTypeConversion  OutDataTypeStr=double
  Demux : Demux  Outputs=3
  Divide : Product  Inputs=*/  OutDataTypeStr=int32
  Mote&PinAreCorrect{0..16} (17 alike) : Logic  AllPortsSameDT=off  OutDataTypeStr=boolean
  MoteID : Constant  Value=0+moteID
  Pin ID : Math  Operator=rem  SaturateOnIntegerOverflow=on
  PinCheck for ADC{0..12} (13 alike) : RelationalOperator  Operator===  OutDataTypeStr=boolean
  PinCheck for DAC0 : RelationalOperator  Operator===  OutDataTypeStr=boolean
  PinCheck for DAC1 : RelationalOperator  Operator===  OutDataTypeStr=boolean
  PinCheck for SerialInput : RelationalOperator  Operator===  OutDataTypeStr=boolean
  PinCheck for SerialOutput : RelationalOperator  Operator===  OutDataTypeStr=boolean
  PinID0 : Constant  Value=0
  PinID1 : Constant
  PinID10 : Constant  Value=10
  PinID11 : Constant  Value=11
  PinID12 : Constant  Value=12
  PinID16-DAC0 : Constant  Value=16
  PinID17-DAC1 : Constant  Value=17
  PinID18-Serial : Constant  Value=18
  PinID19-Serial : Constant  Value=19
  PinID2 : Constant  Value=2
  PinID3 : Constant  Value=3
  PinID4 : Constant  Value=4
  PinID5 : Constant  Value=5
  PinID6 : Constant  Value=6
  PinID7 : Constant  Value=7
  PinID8 : Constant  Value=8
  PinID9 : Constant  Value=9
  Subsystem : Subsystem
  Triggered Subsystem : Subsystem  TreatAsAtomicUnit=on
  Triggered Subsystem1 : Subsystem  TreatAsAtomicUnit=on
  Triggered Subsystem2 : Subsystem  TreatAsAtomicUnit=on
  Triggered Subsystem3 : Subsystem  TreatAsAtomicUnit=on
  Triggered Subsystem4 : Subsystem  TreatAsAtomicUnit=on
  Triggered Subsystem5 : Subsystem  TreatAsAtomicUnit=on
  tIsCrct{0..12,16..17} (15 alike) : Logic  AllPortsSameDT=off  OutDataTypeStr=boolean
  timeIsCrct13 : Logic  AllPortsSameDT=off  OutDataTypeStr=boolean
  timeIsCrct14 : Logic  AllPortsSameDT=off  OutDataTypeStr=boolean
  DAC0 : Outport
  DAC1 : Outport  Port=2
  SerialOutput : Outport  Port=3
  wires:
  Mote&PinAreCorrect11/1 -> tIsCrct11/1
  tIsCrct11/1 -> ADC11-Termin/1
  Mote&PinAreCorrect10/1 -> tIsCrct10/1
  tIsCrct10/1 -> ADC10-Termin/1
  Mote&PinAreCorrect9/1 -> tIsCrct9/1
  tIsCrct9/1 -> ADC9-Termin/1
  tIsCrct8/1 -> ADC8-Termin/1
  tIsCrct7/1 -> ADC7-Termin/1
  tIsCrct5/1 -> Triggered Subsystem1/Trigger  "Enable for ADC5"
  Mote&PinAreCorrect5/1 -> tIsCrct5/1
  tIsCrct6/1 -> ADC6-Termin/1
  tIsCrct4/1 -> ADC4-Termin/1
  tIsCrct3/1 -> ADC3-Termin/1
  Mote&PinAreCorrect2/1 -> tIsCrct2/1
  tIsCrct2/1 -> ADC2-Termin/1
  tIsCrct1/1 -> Triggered Subsystem/Trigger  "Enable for ADC1"
  Mote&PinAreCorrect1/1 -> tIsCrct1/1
  ADC1/1 -> Triggered Subsystem/1(In2)
  tIsCrct0/1 -> ADC0 Sender/Trigger  "Enable for ADC0"
  Mote&PinAreCorrect0/1 -> tIsCrct0/1
  Constant17/1 -> Triggered Subsystem1/1(In2)
  Triggered Subsystem3/1(Out1) -> Data Type Conversion3/1
  Data Type Conversion3/1 -> DAC1/1
  Triggered Subsystem2/1(Out1) -> Data Type Conversion2/1
  Data Type Conversion2/1 -> DAC0/1
  Demux/2 -> Pin ID/1, Divide/1
  ADC0/1 -> ADC0 Sender/1(In2)
  Demux/3 -> Triggered Subsystem2/1(In2), Triggered Subsystem3/1(In2)  "uValue"
  [A] -> Demux/1
  tIsCrct17/1 -> Triggered Subsystem3/Trigger  "Enable for DAC1"
  tIsCrct16/1 -> Triggered Subsystem2/Trigger  "Enable for DAC0"
  Data Type Conversion/1 -> Pin ID/2
  Constant15/1 -> Data Type Conversion/1
  Mote&PinAreCorrect3/1 -> tIsCrct3/1
  Mote&PinAreCorrect4/1 -> tIsCrct4/1
  Mote&PinAreCorrect6/1 -> tIsCrct6/1
  Mote&PinAreCorrect7/1 -> tIsCrct7/1
  Mote&PinAreCorrect8/1 -> tIsCrct8/1
  Mote&PinAreCorrect12/1 -> tIsCrct12/1
  Mote&PinAreCorrect13/1 -> tIsCrct16/1
  MoteID/1 -> Check for moteID/2
  Divide/1 -> Check for moteID/1
  Constant16/1 -> Divide/2
  PinCheck for DAC1/1 -> Mote&PinAreCorrect14/2
  PinCheck for DAC0/1 -> Mote&PinAreCorrect13/2
  PinCheck for ADC12/1 -> Mote&PinAreCorrect12/2
  PinCheck for ADC11/1 -> Mote&PinAreCorrect11/2
  PinCheck for ADC10/1 -> Mote&PinAreCorrect10/2
  PinCheck for ADC9/1 -> Mote&PinAreCorrect9/2
  PinCheck for ADC8/1 -> Mote&PinAreCorrect8/2
  PinCheck for ADC7/1 -> Mote&PinAreCorrect7/2
  PinCheck for ADC6/1 -> Mote&PinAreCorrect6/2
  PinCheck for ADC5/1 -> Mote&PinAreCorrect5/2
  PinCheck for ADC4/1 -> Mote&PinAreCorrect4/2
  PinCheck for ADC3/1 -> Mote&PinAreCorrect3/2
  PinCheck for ADC2/1 -> Mote&PinAreCorrect2/2
  PinCheck for ADC1/1 -> Mote&PinAreCorrect1/2
  PinCheck for ADC0/1 -> Mote&PinAreCorrect0/2
  PinID0/1 -> PinCheck for ADC0/2
  PinID2/1 -> PinCheck for ADC2/2
  PinID3/1 -> PinCheck for ADC3/2
  PinID4/1 -> PinCheck for ADC4/2
  PinID5/1 -> PinCheck for ADC5/2
  PinID6/1 -> PinCheck for ADC6/2
  PinID7/1 -> PinCheck for ADC7/2
  PinID8/1 -> PinCheck for ADC8/2
  PinID10/1 -> PinCheck for ADC10/2
  PinID1/1 -> PinCheck for ADC1/2
  PinID9/1 -> PinCheck for ADC9/2
  PinID11/1 -> PinCheck for ADC11/2
  PinID12/1 -> PinCheck for ADC12/2
  PinID16-DAC0/1 -> PinCheck for DAC0/2
  PinID17-DAC1/1 -> PinCheck for DAC1/2
  Subsystem/1(SerialFrame) -> Triggered Subsystem5/1(SerialDataToSend)
  Demux/1 -> tIsCrct0/2, tIsCrct1/2, tIsCrct2/2, tIsCrct3/2, tIsCrct4/2, tIsCrct5/2, tIsCrct6/2, tIsCrct7/2, tIsCrct8/2, tIsCrct9/2, tIsCrct10/2, tIsCrct11/2, tIsCrct12/2, tIsCrct16/2, timeIsCrct14/1, timeIsCrct13/1, tIsCrct17/1  "TimeIsCorrect"
  PinID18-Serial/1 -> PinCheck for SerialInput/2
  [SerialData] -> Triggered Subsystem4/1(RecivedSD)
  timeIsCrct13/1 -> Triggered Subsystem4/Trigger
  Mote&PinAreCorrect14/1 -> tIsCrct17/2  "TimeIsCorrect"
  Triggered Subsystem4/1(SDToApplay) -> SerialOutput/1
  tIsCrct12/1 -> ADC12-Termin/1
  Pin ID/1 -> PinCheck for ADC0/1, PinCheck for ADC1/1, PinCheck for ADC2/1, PinCheck for SerialOutput/1, PinCheck for SerialInput/1, PinCheck for DAC1/1, PinCheck for DAC0/1, PinCheck for ADC12/1, PinCheck for ADC11/1, PinCheck for ADC10/1, PinCheck for ADC9/1, PinCheck for ADC8/1, PinCheck for ADC7/1, PinCheck for ADC6/1, PinCheck for ADC5/1, PinCheck for ADC4/1, PinCheck for ADC3/1  "Pin number"
  Mote&PinAreCorrect15/1 -> timeIsCrct13/2
  Check for moteID/1 -> Mote&PinAreCorrect1/1, Mote&PinAreCorrect13/1, Mote&PinAreCorrect14/1, Mote&PinAreCorrect16/1, Mote&PinAreCorrect15/1, Mote&PinAreCorrect12/1, Mote&PinAreCorrect11/1, Mote&PinAreCorrect10/1, Mote&PinAreCorrect9/1, Mote&PinAreCorrect8/1, Mote&PinAreCorrect7/1, Mote&PinAreCorrect6/1, Mote&PinAreCorrect5/1, Mote&PinAreCorrect4/1, Mote&PinAreCorrect3/1, Mote&PinAreCorrect2/1, Mote&PinAreCorrect0/1  "Is message related to this mote"
  PinID19-Serial/1 -> PinCheck for SerialOutput/2
  PinCheck for SerialOutput/1 -> Mote&PinAreCorrect16/2
  Mote&PinAreCorrect16/1 -> timeIsCrct14/2
  timeIsCrct14/1 -> Triggered Subsystem5/Trigger
  SerialInput/1 -> Data Type Conversion1/1
  Data Type Conversion1/1 -> Subsystem/1(SerialData)
  PinCheck for SerialInput/1 -> Mote&PinAreCorrect15/2

== system WaterTank_10Tanks_Model/GISOO-Simulation Environment/SkyMote5 ==
  note: Interface Identifier
  ADC0 : Inport
  ADC1 : Inport  Port=2
  SerialInput : Inport  Port=3
  ADC0 Sender : Subsystem  TreatAsAtomicUnit=on
  ADC10-Termin : Terminator
  ADC11-Termin : Terminator
  ADC12-Termin : Terminator
  ADC2-Termin : Terminator
  ADC3-Termin : Terminator
  ADC4-Termin : Terminator
  ADC6-Termin : Terminator
  ADC7-Termin : Terminator
  ADC8-Termin : Terminator
  ADC9-Termin : Terminator
  Check for moteID : RelationalOperator  Operator===  OutDataTypeStr=boolean
  Constant15 : Constant  Value=100
  Constant16 : Constant  Value=100
  Constant17 : Constant  Value=5
  Data Type Conversion : DataTypeConversion  OutDataTypeStr=uint32
  Data Type Conversion1 : DataTypeConversion  OutDataTypeStr=uint32
  Data Type Conversion2 : DataTypeConversion  OutDataTypeStr=double
  Data Type Conversion3 : DataTypeConversion  OutDataTypeStr=double
  Demux : Demux  Outputs=3
  Divide : Product  Inputs=*/  OutDataTypeStr=int32
  Mote&PinAreCorrect{0..16} (17 alike) : Logic  AllPortsSameDT=off  OutDataTypeStr=boolean
  MoteID : Constant  Value=0+moteID
  Pin ID : Math  Operator=rem  SaturateOnIntegerOverflow=on
  PinCheck for ADC{0..12} (13 alike) : RelationalOperator  Operator===  OutDataTypeStr=boolean
  PinCheck for DAC0 : RelationalOperator  Operator===  OutDataTypeStr=boolean
  PinCheck for DAC1 : RelationalOperator  Operator===  OutDataTypeStr=boolean
  PinCheck for SerialInput : RelationalOperator  Operator===  OutDataTypeStr=boolean
  PinCheck for SerialOutput : RelationalOperator  Operator===  OutDataTypeStr=boolean
  PinID0 : Constant  Value=0
  PinID1 : Constant
  PinID10 : Constant  Value=10
  PinID11 : Constant  Value=11
  PinID12 : Constant  Value=12
  PinID16-DAC0 : Constant  Value=16
  PinID17-DAC1 : Constant  Value=17
  PinID18-Serial : Constant  Value=18
  PinID19-Serial : Constant  Value=19
  PinID2 : Constant  Value=2
  PinID3 : Constant  Value=3
  PinID4 : Constant  Value=4
  PinID5 : Constant  Value=5
  PinID6 : Constant  Value=6
  PinID7 : Constant  Value=7
  PinID8 : Constant  Value=8
  PinID9 : Constant  Value=9
  Subsystem : Subsystem
  Triggered Subsystem : Subsystem  TreatAsAtomicUnit=on
  Triggered Subsystem1 : Subsystem  TreatAsAtomicUnit=on
  Triggered Subsystem2 : Subsystem  TreatAsAtomicUnit=on
  Triggered Subsystem3 : Subsystem  TreatAsAtomicUnit=on
  Triggered Subsystem4 : Subsystem  TreatAsAtomicUnit=on
  Triggered Subsystem5 : Subsystem  TreatAsAtomicUnit=on
  tIsCrct{0..12,16..17} (15 alike) : Logic  AllPortsSameDT=off  OutDataTypeStr=boolean
  timeIsCrct13 : Logic  AllPortsSameDT=off  OutDataTypeStr=boolean
  timeIsCrct14 : Logic  AllPortsSameDT=off  OutDataTypeStr=boolean
  DAC0 : Outport
  DAC1 : Outport  Port=2
  SerialOutput : Outport  Port=3
  wires:
  PinCheck for SerialInput/1 -> Mote&PinAreCorrect15/2
  Data Type Conversion1/1 -> Subsystem/1(SerialData)
  SerialInput/1 -> Data Type Conversion1/1
  timeIsCrct14/1 -> Triggered Subsystem5/Trigger
  Mote&PinAreCorrect16/1 -> timeIsCrct14/2
  PinCheck for SerialOutput/1 -> Mote&PinAreCorrect16/2
  PinID19-Serial/1 -> PinCheck for SerialOutput/2
  Check for moteID/1 -> Mote&PinAreCorrect0/1, Mote&PinAreCorrect2/1, Mote&PinAreCorrect3/1, Mote&PinAreCorrect4/1, Mote&PinAreCorrect5/1, Mote&PinAreCorrect6/1, Mote&PinAreCorrect7/1, Mote&PinAreCorrect8/1, Mote&PinAreCorrect9/1, Mote&PinAreCorrect10/1, Mote&PinAreCorrect11/1, Mote&PinAreCorrect12/1, Mote&PinAreCorrect15/1, Mote&PinAreCorrect16/1, Mote&PinAreCorrect14/1, Mote&PinAreCorrect13/1, Mote&PinAreCorrect1/1  "Is message related to this mote"
  Mote&PinAreCorrect15/1 -> timeIsCrct13/2
  Pin ID/1 -> PinCheck for ADC3/1, PinCheck for ADC4/1, PinCheck for ADC5/1, PinCheck for ADC6/1, PinCheck for ADC7/1, PinCheck for ADC8/1, PinCheck for ADC9/1, PinCheck for ADC10/1, PinCheck for ADC11/1, PinCheck for ADC12/1, PinCheck for DAC0/1, PinCheck for DAC1/1, PinCheck for SerialInput/1, PinCheck for SerialOutput/1, PinCheck for ADC2/1, PinCheck for ADC1/1, PinCheck for ADC0/1  "Pin number"
  tIsCrct12/1 -> ADC12-Termin/1
  Triggered Subsystem4/1(SDToApplay) -> SerialOutput/1
  Mote&PinAreCorrect14/1 -> tIsCrct17/2  "TimeIsCorrect"
  timeIsCrct13/1 -> Triggered Subsystem4/Trigger
  [SerialData] -> Triggered Subsystem4/1(RecivedSD)
  PinID18-Serial/1 -> PinCheck for SerialInput/2
  Demux/1 -> tIsCrct17/1, timeIsCrct13/1, timeIsCrct14/1, tIsCrct16/2, tIsCrct12/2, tIsCrct11/2, tIsCrct10/2, tIsCrct9/2, tIsCrct8/2, tIsCrct7/2, tIsCrct6/2, tIsCrct5/2, tIsCrct4/2, tIsCrct3/2, tIsCrct2/2, tIsCrct1/2, tIsCrct0/2  "TimeIsCorrect"
  Subsystem/1(SerialFrame) -> Triggered Subsystem5/1(SerialDataToSend)
  PinID17-DAC1/1 -> PinCheck for DAC1/2
  PinID16-DAC0/1 -> PinCheck for DAC0/2
  PinID12/1 -> PinCheck for ADC12/2
  PinID11/1 -> PinCheck for ADC11/2
  PinID9/1 -> PinCheck for ADC9/2
  PinID1/1 -> PinCheck for ADC1/2
  PinID10/1 -> PinCheck for ADC10/2
  PinID8/1 -> PinCheck for ADC8/2
  PinID7/1 -> PinCheck for ADC7/2
  PinID6/1 -> PinCheck for ADC6/2
  PinID5/1 -> PinCheck for ADC5/2
  PinID4/1 -> PinCheck for ADC4/2
  PinID3/1 -> PinCheck for ADC3/2
  PinID2/1 -> PinCheck for ADC2/2
  PinID0/1 -> PinCheck for ADC0/2
  PinCheck for ADC0/1 -> Mote&PinAreCorrect0/2
  PinCheck for ADC1/1 -> Mote&PinAreCorrect1/2
  PinCheck for ADC2/1 -> Mote&PinAreCorrect2/2
  PinCheck for ADC3/1 -> Mote&PinAreCorrect3/2
  PinCheck for ADC4/1 -> Mote&PinAreCorrect4/2
  PinCheck for ADC5/1 -> Mote&PinAreCorrect5/2
  PinCheck for ADC6/1 -> Mote&PinAreCorrect6/2
  PinCheck for ADC7/1 -> Mote&PinAreCorrect7/2
  PinCheck for ADC8/1 -> Mote&PinAreCorrect8/2
  PinCheck for ADC9/1 -> Mote&PinAreCorrect9/2
  PinCheck for ADC10/1 -> Mote&PinAreCorrect10/2
  PinCheck for ADC11/1 -> Mote&PinAreCorrect11/2
  PinCheck for ADC12/1 -> Mote&PinAreCorrect12/2
  PinCheck for DAC0/1 -> Mote&PinAreCorrect13/2
  PinCheck for DAC1/1 -> Mote&PinAreCorrect14/2
  Constant16/1 -> Divide/2
  Divide/1 -> Check for moteID/1
  MoteID/1 -> Check for moteID/2
  Mote&PinAreCorrect13/1 -> tIsCrct16/1
  Mote&PinAreCorrect12/1 -> tIsCrct12/1
  Mote&PinAreCorrect8/1 -> tIsCrct8/1
  Mote&PinAreCorrect7/1 -> tIsCrct7/1
  Mote&PinAreCorrect6/1 -> tIsCrct6/1
  Mote&PinAreCorrect4/1 -> tIsCrct4/1
  Mote&PinAreCorrect3/1 -> tIsCrct3/1
  Constant15/1 -> Data Type Conversion/1
  Data Type Conversion/1 -> Pin ID/2
  tIsCrct16/1 -> Triggered Subsystem2/Trigger  "Enable for DAC0"
  tIsCrct17/1 -> Triggered Subsystem3/Trigger  "Enable for DAC1"
  [A] -> Demux/1
  Demux/3 -> Triggered Subsystem3/1(In2), Triggered Subsystem2/1(In2)  "uValue"
  ADC0/1 -> ADC0 Sender/1(In2)
  Demux/2 -> Divide/1, Pin ID/1
  Data Type Conversion2/1 -> DAC0/1
  Triggered Subsystem2/1(Out1) -> Data Type Conversion2/1
  Data Type Conversion3/1 -> DAC1/1
  Triggered Subsystem3/1(Out1) -> Data Type Conversion3/1
  Constant17/1 -> Triggered Subsystem1/1(In2)
  Mote&PinAreCorrect0/1 -> tIsCrct0/1
  tIsCrct0/1 -> ADC0 Sender/Trigger  "Enable for ADC0"
  ADC1/1 -> Triggered Subsystem/1(In2)
  Mote&PinAreCorrect1/1 -> tIsCrct1/1
  tIsCrct1/1 -> Triggered Subsystem/Trigger  "Enable for ADC1"
  tIsCrct2/1 -> ADC2-Termin/1
  Mote&PinAreCorrect2/1 -> tIsCrct2/1
  tIsCrct3/1 -> ADC3-Termin/1
  tIsCrct4/1 -> ADC4-Termin/1
  tIsCrct6/1 -> ADC6-Termin/1
  Mote&PinAreCorrect5/1 -> tIsCrct5/1
  tIsCrct5/1 -> Triggered Subsystem1/Trigger  "Enable for ADC5"
  tIsCrct7/1 -> ADC7-Termin/1
  tIsCrct8/1 -> ADC8-Termin/1
  tIsCrct9/1 -> ADC9-Termin/1
  Mote&PinAreCorrect9/1 -> tIsCrct9/1
  tIsCrct10/1 -> ADC10-Termin/1
  Mote&PinAreCorrect10/1 -> tIsCrct10/1
  tIsCrct11/1 -> ADC11-Termin/1
  Mote&PinAreCorrect11/1 -> tIsCrct11/1
